simulink model "Ikeda_n"  (R2018b)
settings: Solver=ode4  StartTime=0.0  StopTime=6e6  FixedStep=1  RelTol=1e-3
undefined symbols (not defined in the file or in its folder): const
libraries: simulink x1
settings Model: Creator=DD  LastModifiedBy=DD

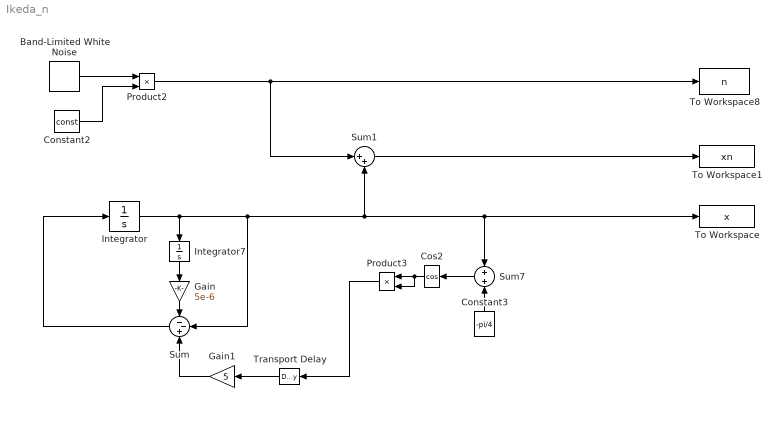
== system Ikeda_n ==
  Band-Limited White Noise : simulink/Sources/Band-Limited White Noise  Cov=[0.1]  Ts=1  seed=[23341]
  Constant2 : Constant  Value=const
  Constant3 : Constant  Value=-pi/4
  Cos2 : Trigonometry  Operator=cos
  Gain : Gain  Gain=5e-6
  Gain1 : Gain  Gain=5
  Integrator : Integrator  InitialCondition=0.1
  Integrator7 : Integrator
  Product2 : Product
  Product3 : Product
  Sum : Sum  Inputs=--+
  Sum1 : Sum  Inputs=|++
  Sum7 : Sum
  To Workspace : ToWorkspace  VariableName=x  SampleTime=-1
  To Workspace1 : ToWorkspace  VariableName=xn  SampleTime=-1
  To Workspace8 : ToWorkspace  VariableName=n  SampleTime=-1
  Transport Delay : TransportDelay  DelayTime=1200  BufferSize=100000
  wires:
  Constant3/1 -> Sum7/2
  Sum7/1 -> Cos2/1
  Integrator/1 -> Sum/2, Sum1/2, To Workspace/1, Sum7/1, Integrator7/1
  Product3/1 -> Transport Delay/1
  Cos2/1 -> Product3/2, Product3/1
  Gain/1 -> Sum/1
  Product2/1 -> Sum1/1, To Workspace8/1
  Constant2/1 -> Product2/2
  Sum/1 -> Integrator/1
  Gain1/1 -> Sum/3
  Transport Delay/1 -> Gain1/1
  Band-Limited White Noise/1 -> Product2/1
  Integrator7/1 -> Gain/1
  Sum1/1 -> To Workspace1/1
